simulink model "tempreature"  (R2021b)
settings: Solver=VariableStepAuto  StartTime=0.0  StopTime=20.0  RelTol=1e-3
libraries: fuzblock x1
settings Model: Creator=Mahban  LastModifiedBy=Mahban

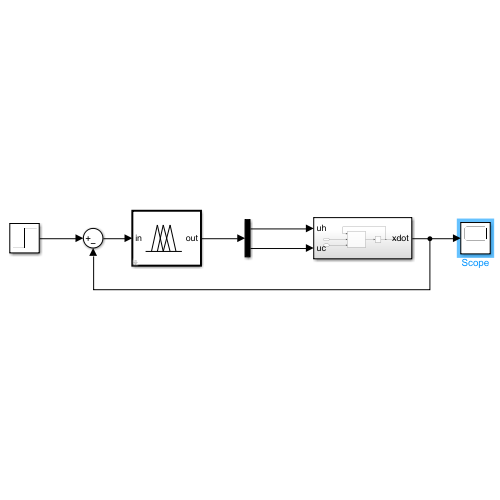
[thumbnail: Simulink's stored preview of the top-level diagram]
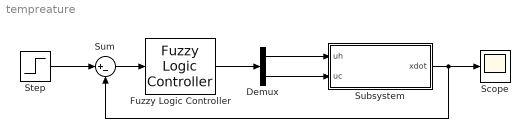
== system tempreature ==
  Demux : Demux  Outputs=2
  Fuzzy Logic Controller : fuzblock/Fuzzy Logic  Controller  FIS=myFIS  OutputSampleNumber=101  DataType=double  FuzzifiedInputs=off  RuleFiringStrengths=off  RuleOutputs=off  AggregatedOutputs=off  SimulateUsing=Interpreted execution  OutOfRangeInputValueMessage=warning  NoRuleFiredMessage=warning  EmptyOutputFuzzySetMessage=warning
  Scope : Scope
  Step : Step  SampleTime=0
  Subsystem : Subsystem
  Sum : Sum  Inputs=|+-
  wires:
  Fuzzy Logic Controller/1 -> Demux/1
  Subsystem/1(xdot) -> Sum/2, Scope/1
  Demux/1 -> Subsystem/1(uh)
  Demux/2 -> Subsystem/2(uc)
  Step/1 -> Sum/1
  Sum/1 -> Fuzzy Logic Controller/1

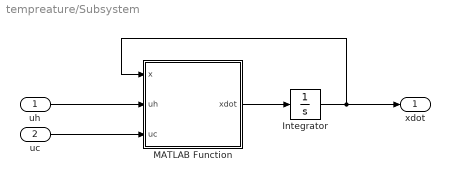
== system tempreature/Subsystem ==
  uh : Inport
  uc : Inport  Port=2
  Integrator : Integrator
  MATLAB Function : MATLAB Function  TreatAsAtomicUnit=on
  xdot : Outport
  wires:
  uh/1 -> MATLAB Function/2(uh)
  uc/1 -> MATLAB Function/3(uc)
  MATLAB Function/1(xdot) -> Integrator/1
  Integrator/1 -> MATLAB Function/1(x), xdot/1

== matlab function tempreature/Subsystem/MATLAB Function ==
  data: x input; xdot output; uh input; uc input
function xdot = fcn(x,uh,uc)

xdot=-(x-16)+2*uh-2*uc;
